simulink model "L1HeadingController"  (R2015a)
settings: Solver=ode4  StartTime=0.0  StopTime=10.0  FixedStep=0.01  RelTol=1e-3
undefined symbols (not defined in the file): a1, a2, delta_rate_limit, Pb_yaw, proj_omega_0_yaw, proj_omega_bound_yaw, proj_omega_center_yaw, proj_omega_eps_yaw, proj_sigma_0_yaw, proj_sigma_bound_yaw, proj_sigma_center_yaw, proj_sigma_eps_yaw, proj_theta_0_yaw, proj_theta_bound_yaw, proj_theta_center_yaw, proj_theta_eps_yaw, T, theta_1, Ts, Ts_yaw_L1
libraries: vrlib x6, simulink x2
settings Model: Creator=s120949  LastModifiedBy=s120949
settings OptimizationCC: OptimizeModelRefInitCode=on  LifeSpan=1
settings RTWCC: SystemTargetFile=ert.tlc  GenCodeOnly=on  TemplateMakefile=ert_default_tmf  Description=Embedded Coder  BuildConfiguration=Faster Runs
settings CodeAppCC: IgnoreCustomStorageClasses=off  SignalNamingRule=Custom
settings ERTTargetCC: ParMdlRefBuildCompliant=on  CompOptLevelCompliant=on  ConcurrentExecutionCompliant=on  ERTFirstTimeCompliant=on  SupportContinuousTime=off  SupportVariableSizeSignals=off  ModelStepFunctionPrototypeControlCompliant=on  CPPClassGenCompliant=on  InlinedParameterPlacement=Hierarchical  ERTCustomFileTemplate=example_file_process.tlc  ConvertIfToSwitch=on

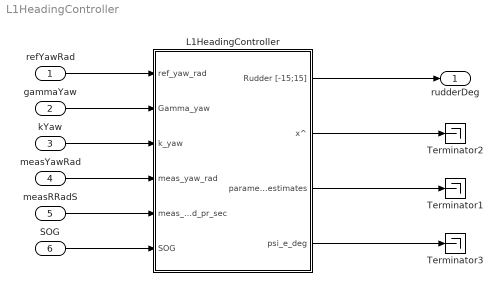
== system L1HeadingController ==
  refYawRad : Inport
  gammaYaw : Inport  Port=2
  kYaw : Inport  Port=3
  measYawRad : Inport  Port=4
  measRRadS : Inport  Port=5
  SOG : Inport  Port=6
  L1HeadingController : Subsystem  TreatAsAtomicUnit=on
      settings: RTWSystemCode=Nonreusable function
  Terminator1 : Terminator
  Terminator2 : Terminator
  Terminator3 : Terminator
  rudderDeg : Outport
  wires:
  refYawRad/1 -> L1HeadingController/1(ref_yaw_rad)
  L1HeadingController/1(Rudder [-15;15]) -> rudderDeg/1
  gammaYaw/1 -> L1HeadingController/2(Gamma_yaw)
  kYaw/1 -> L1HeadingController/3(k_yaw)
  measYawRad/1 -> L1HeadingController/4(meas_yaw_rad)
  measRRadS/1 -> L1HeadingController/5(meas_R_rad_pr_sec)
  SOG/1 -> L1HeadingController/6(SOG)
  L1HeadingController/2(x^) -> Terminator2/1
  L1HeadingController/4(psi_e_deg) -> Terminator3/1
  L1HeadingController/3(parameter_estimates) -> Terminator1/1

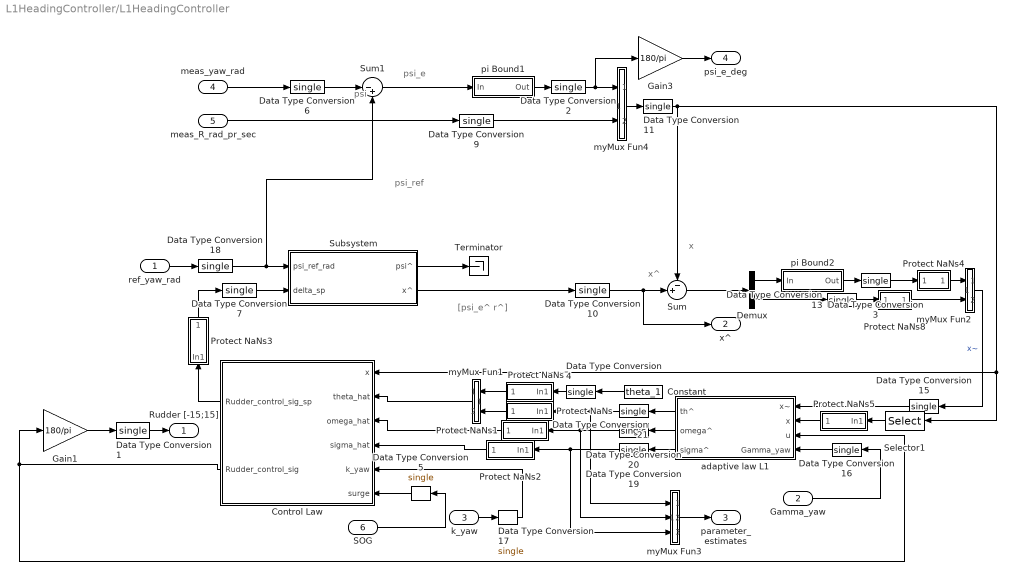
== system L1HeadingController/L1HeadingController ==
  note: x^
  note: [psi_e^ r^]
  note: x
  note: psi
  note: psi_ref
  note: psi_e
  ref_yaw_rad : Inport
  Gamma_yaw : Inport  Port=2
  k_yaw : Inport  Port=3
  meas_yaw_rad : Inport  Port=4
  meas_R_rad_pr_sec : Inport  Port=5
  SOG : Inport  Port=6
  Constant : Constant  Value=theta_1  SampleTime=Ts_yaw_L1
  Control Law : Subsystem
  Data Type Conversion{1..7,9..11,13,15..21} (18 alike) : DataTypeConversion  OutDataTypeStr=single
  Demux : Demux  Outputs=2
  Gain1 : Gain  Gain=180/pi
  Gain3 : Gain  Gain=180/pi
  Protect NaNs : Subsystem
  Protect NaNs1 : Subsystem
  Protect NaNs2 : Subsystem
  Protect NaNs3 : Subsystem
  Protect NaNs4 : Subsystem
  Protect NaNs5 : Subsystem
  Protect NaNs7 : Subsystem
  Protect NaNs8 : Subsystem
  Selector1 : Selector  InputPortWidth=2  Indices=2
  Subsystem : Subsystem
  Sum : Sum  Inputs=-+|
  Sum1 : Sum  Inputs=|-+
  Terminator : Terminator
  adaptive law L1 : Subsystem
  myMux Fun1 : MATLAB Function  TreatAsAtomicUnit=on
  myMux Fun2 : MATLAB Function  TreatAsAtomicUnit=on
  myMux Fun3 : MATLAB Function  TreatAsAtomicUnit=on
  myMux Fun4 : MATLAB Function  TreatAsAtomicUnit=on
  pi Bound1 : Subsystem  AncestorBlock=aerosimlib/Math/pi Bound  mask(pi bound){}
      mask help: Bounds the input angle to [-pi, pi]. When -pi bound is exceeded the output wraps back to pi; when the pi bound is exceeded the output wraps back to -pi.
      mask Help:
      | Bounds the input angle to [-pi, pi]. When -pi bound is exceeded the output wraps back to pi; when the pi bound is exceeded the output wraps back to -pi.
      | <P><B>Input:</B> any angle in radians, from -Inf to Inf;</P>
      | <P><B>Output:</B> an angle in radians between -pi and pi.</P>
  pi Bound2 : Subsystem  AncestorBlock=aerosimlib/Math/pi Bound  mask(pi bound){}
      mask help: Bounds the input angle to [-pi, pi]. When -pi bound is exceeded the output wraps back to pi; when the pi bound is exceeded the output wraps back to -pi.
      mask Help:
      | Bounds the input angle to [-pi, pi]. When -pi bound is exceeded the output wraps back to pi; when the pi bound is exceeded the output wraps back to -pi.
      | <P><B>Input:</B> any angle in radians, from -Inf to Inf;</P>
      | <P><B>Output:</B> an angle in radians between -pi and pi.</P>
  Rudder [-15;15] : Outport
  x^ : Outport  Port=2
  parameter_estimates : Outport  Port=3
  psi_e_deg : Outport  Port=4
  wires:
  Gamma_yaw/1 -> Data Type Conversion16/1
  k_yaw/1 -> Data Type Conversion17/1
  adaptive law L1/3(sigma^) -> Data Type Conversion19/1
  adaptive law L1/2(omega^) -> Data Type Conversion20/1
  ref_yaw_rad/1 -> Data Type Conversion18/1
  Control Law/2(Rudder_control_sig) -> adaptive law L1/3(u), Gain1/1
  adaptive law L1/1(th^) -> Data Type Conversion21/1
  Control Law/1(Rudder_control_sig_sp) -> Protect NaNs3/1(In1)
  meas_yaw_rad/1 -> Data Type Conversion6/1
  meas_R_rad_pr_sec/1 -> Data Type Conversion9/1
  Sum/1 -> Demux/1
  Demux/1 -> pi Bound2/1(In)
  Demux/2 -> Data Type Conversion13/1
  pi Bound2/1(Out) -> Data Type Conversion3/1
  myMux Fun2/1(y) -> Data Type Conversion15/1  "x~"
  Subsystem/2(x^) -> Data Type Conversion10/1
  pi Bound1/1(Out) -> Data Type Conversion2/1
  myMux Fun4/1(y) -> Data Type Conversion11/1
  Sum1/1 -> pi Bound1/1(In)
  Subsystem/1(psi^) -> Terminator/1
  Data Type Conversion1/1 -> Rudder [-15;15]/1
  Data Type Conversion6/1 -> Sum1/1
  Data Type Conversion9/1 -> myMux Fun4/2(u2)
  Data Type Conversion10/1 -> Sum/2, x^/1
  Data Type Conversion11/1 -> Sum/1, Control Law/1(x), Selector1/1
  Data Type Conversion13/1 -> Protect NaNs8/1(In1)
  Data Type Conversion15/1 -> adaptive law L1/1(x~)
  Data Type Conversion16/1 -> adaptive law L1/4(Gamma_yaw)
  Data Type Conversion17/1 -> Control Law/5(k_yaw)
  Data Type Conversion18/1 -> Subsystem/1(psi_ref_rad), Sum1/2
  Data Type Conversion7/1 -> Subsystem/2(delta_sp)
  Data Type Conversion19/1 -> myMux Fun3/3(u3), Protect NaNs2/1(In1)
  Data Type Conversion20/1 -> myMux Fun3/2(u2), Protect NaNs1/1(In1)
  Data Type Conversion2/1 -> myMux Fun4/1(u1), Gain3/1
  Gain3/1 -> psi_e_deg/1
  Gain1/1 -> Data Type Conversion1/1
  Selector1/1 -> Protect NaNs5/1(In1)
  Data Type Conversion21/1 -> myMux Fun3/1(u1), Protect NaNs/1(In1)
  Data Type Conversion4/1 -> Protect NaNs7/1(In1)
  myMux Fun1/1(y) -> Control Law/2(theta_hat)
  Constant/1 -> Data Type Conversion4/1
  myMux Fun3/1(y) -> parameter_estimates/1
  Protect NaNs/1(Out1) -> myMux Fun1/2(u2)
  Protect NaNs1/1(Out1) -> Control Law/3(omega_hat)
  Protect NaNs2/1(Out1) -> Control Law/4(sigma_hat)
  Protect NaNs3/1(Out1) -> Data Type Conversion7/1
  Protect NaNs7/1(Out1) -> myMux Fun1/1(u1)
  Protect NaNs5/1(Out1) -> adaptive law L1/2(x)
  Protect NaNs4/1(Out1) -> myMux Fun2/1(u1)
  Protect NaNs8/1(Out1) -> myMux Fun2/2(u2)
  Data Type Conversion3/1 -> Protect NaNs4/1(In1)
  Data Type Conversion5/1 -> Control Law/6(surge)
  SOG/1 -> Data Type Conversion5/1

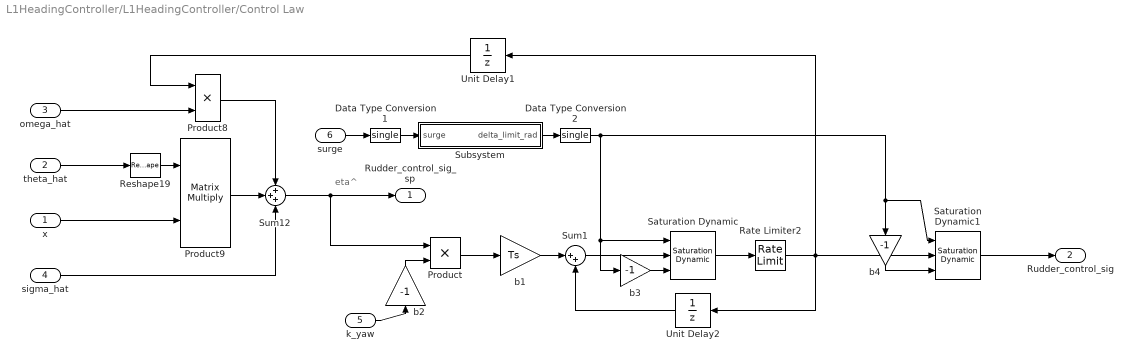
== system L1HeadingController/L1HeadingController/Control Law ==
  note: eta^
  x : Inport
  theta_hat : Inport  Port=2
  omega_hat : Inport  Port=3
  sigma_hat : Inport  Port=4
  k_yaw : Inport  Port=5
  surge : Inport  Port=6
  Data Type Conversion1 : DataTypeConversion  OutDataTypeStr=single
  Data Type Conversion2 : DataTypeConversion  OutDataTypeStr=single
  Product : Product  RndMeth=Zero
  Product8 : Product  RndMeth=Zero
  Product9 : Product  Multiplication=Matrix(*)  RndMeth=Zero
  Rate Limiter2 : RateLimiter  RisingSlewLimit=delta_rate_limit  FallingSlewLimit=-delta_rate_limit  SampleTimeMode=inherited
  Reshape19 : Reshape  OutputDimensionality=Row vector (2-D)
  Saturation Dynamic : simulink/Discontinuities/Saturation Dynamic  OutMin=[]  OutMax=[]  OutDataTypeStr=Inherit: Same as second input  OutDataType=fixdt(1, 16)  OutScaling=2^-10  DoSatur=off
  Saturation Dynamic1 : simulink/Discontinuities/Saturation Dynamic  OutMin=[]  OutMax=[]  OutDataTypeStr=Inherit: Same as second input  OutDataType=fixdt(1, 16)  OutScaling=2^-10  DoSatur=off
  Subsystem : Subsystem
  Sum1 : Sum  Inputs=|++
  Sum12 : Sum  Inputs=+++
  Unit Delay1 : UnitDelay  SampleTime=Ts
  Unit Delay2 : UnitDelay  SampleTime=Ts
  b1 : Gain  Gain=Ts  SampleTime=Ts
  b2 : Gain  Gain=-1
  b3 : Gain  Gain=-1
  b4 : Gain  Gain=-1
  Rudder_control_sig_sp : Outport
  Rudder_control_sig : Outport  Port=2
  wires:
  k_yaw/1 -> b2/1
  b2/1 -> Product/2
  Unit Delay1/1 -> Product8/1
  Product/1 -> b1/1
  Sum12/1 -> Rudder_control_sig_sp/1, Product/1
  sigma_hat/1 -> Sum12/3
  Product8/1 -> Sum12/1
  Product9/1 -> Sum12/2
  x/1 -> Product9/2
  Reshape19/1 -> Product9/1
  theta_hat/1 -> Reshape19/1
  omega_hat/1 -> Product8/2
  Sum1/1 -> Saturation Dynamic/2
  Saturation Dynamic/1 -> Rate Limiter2/1
  b1/1 -> Sum1/1
  Subsystem/1(delta_limit_rad) -> Data Type Conversion2/1
  b3/1 -> Saturation Dynamic/3
  surge/1 -> Data Type Conversion1/1
  Rate Limiter2/1 -> Unit Delay1/1, Saturation Dynamic1/2, Unit Delay2/1
  Unit Delay2/1 -> Sum1/2
  Saturation Dynamic1/1 -> Rudder_control_sig/1
  b4/1 -> Saturation Dynamic1/3
  Data Type Conversion1/1 -> Subsystem/1(surge)
  Data Type Conversion2/1 -> Saturation Dynamic/1, b3/1, Saturation Dynamic1/1, b4/1

== system L1HeadingController/L1HeadingController/Protect NaNs ==
  In1 : Inport
  Integer Delay3 : Delay  DelayLength=1  InputProcessing=Inherited  SampleTime=T
  Relational Operator2 : RelationalOperator  Operator===  OutDataTypeStr=uint(8)
  Switch3 : Switch  Criteria=u2 > Threshold  Threshold=0.3  SampleTime=.01
  Out1 : Outport
  wires:
  Integer Delay3/1 -> Switch3/3
  Switch3/1 -> Out1/1, Integer Delay3/1
  In1/1 -> Relational Operator2/2, Relational Operator2/1, Switch3/1
  Relational Operator2/1 -> Switch3/2

== system L1HeadingController/L1HeadingController/Protect NaNs1 ==
  In1 : Inport
  Integer Delay3 : Delay  DelayLength=1  InputProcessing=Inherited  SampleTime=T
  Relational Operator2 : RelationalOperator  Operator===  OutDataTypeStr=uint(8)
  Switch3 : Switch  Criteria=u2 > Threshold  Threshold=0.3  SampleTime=.01
  Out1 : Outport
  wires:
  Relational Operator2/1 -> Switch3/2
  In1/1 -> Switch3/1, Relational Operator2/1, Relational Operator2/2
  Switch3/1 -> Integer Delay3/1, Out1/1
  Integer Delay3/1 -> Switch3/3

== system L1HeadingController/L1HeadingController/Protect NaNs2 ==
  In1 : Inport
  Integer Delay3 : Delay  DelayLength=1  InputProcessing=Inherited  SampleTime=T
  Relational Operator2 : RelationalOperator  Operator===  OutDataTypeStr=uint(8)
  Switch3 : Switch  Criteria=u2 > Threshold  Threshold=0.3  SampleTime=.01
  Out1 : Outport
  wires:
  Integer Delay3/1 -> Switch3/3
  Switch3/1 -> Out1/1, Integer Delay3/1
  In1/1 -> Relational Operator2/2, Relational Operator2/1, Switch3/1
  Relational Operator2/1 -> Switch3/2

== system L1HeadingController/L1HeadingController/Protect NaNs3 ==
  In1 : Inport
  Integer Delay3 : Delay  DelayLength=1  InputProcessing=Inherited  SampleTime=T
  Relational Operator2 : RelationalOperator  Operator===  OutDataTypeStr=uint(8)
  Switch3 : Switch  Criteria=u2 > Threshold  Threshold=0.3  SampleTime=.01
  Out1 : Outport
  wires:
  Relational Operator2/1 -> Switch3/2
  In1/1 -> Switch3/1, Relational Operator2/1, Relational Operator2/2
  Switch3/1 -> Integer Delay3/1, Out1/1
  Integer Delay3/1 -> Switch3/3

== system L1HeadingController/L1HeadingController/Protect NaNs4 ==
  In1 : Inport
  Integer Delay3 : Delay  DelayLength=1  InputProcessing=Inherited  SampleTime=T
  Relational Operator2 : RelationalOperator  Operator===  OutDataTypeStr=uint(8)
  Switch3 : Switch  Criteria=u2 > Threshold  Threshold=0.3  SampleTime=.01
  Out1 : Outport
  wires:
  Integer Delay3/1 -> Switch3/3
  Switch3/1 -> Out1/1, Integer Delay3/1
  In1/1 -> Relational Operator2/2, Relational Operator2/1, Switch3/1
  Relational Operator2/1 -> Switch3/2

== system L1HeadingController/L1HeadingController/Protect NaNs5 ==
  In1 : Inport
  Integer Delay3 : Delay  DelayLength=1  InputProcessing=Inherited  SampleTime=T
  Relational Operator2 : RelationalOperator  Operator===  OutDataTypeStr=uint(8)
  Switch3 : Switch  Criteria=u2 > Threshold  Threshold=0.3  SampleTime=.01
  Out1 : Outport
  wires:
  Relational Operator2/1 -> Switch3/2
  In1/1 -> Switch3/1, Relational Operator2/1, Relational Operator2/2
  Switch3/1 -> Integer Delay3/1, Out1/1
  Integer Delay3/1 -> Switch3/3

== system L1HeadingController/L1HeadingController/Protect NaNs7 ==
  In1 : Inport
  Integer Delay3 : Delay  DelayLength=1  InputProcessing=Inherited  SampleTime=T
  Relational Operator2 : RelationalOperator  Operator===  OutDataTypeStr=uint(8)
  Switch3 : Switch  Criteria=u2 > Threshold  Threshold=0.3  SampleTime=.01
  Out1 : Outport
  wires:
  Relational Operator2/1 -> Switch3/2
  In1/1 -> Switch3/1, Relational Operator2/1, Relational Operator2/2
  Switch3/1 -> Integer Delay3/1, Out1/1
  Integer Delay3/1 -> Switch3/3

== system L1HeadingController/L1HeadingController/Protect NaNs8 ==
  In1 : Inport
  Integer Delay3 : Delay  DelayLength=1  InputProcessing=Inherited  SampleTime=T
  Relational Operator2 : RelationalOperator  Operator===  OutDataTypeStr=uint(8)
  Switch3 : Switch  Criteria=u2 > Threshold  Threshold=0.3  SampleTime=.01
  Out1 : Outport
  wires:
  Relational Operator2/1 -> Switch3/2
  In1/1 -> Switch3/1, Relational Operator2/1, Relational Operator2/2
  Switch3/1 -> Integer Delay3/1, Out1/1
  Integer Delay3/1 -> Switch3/3

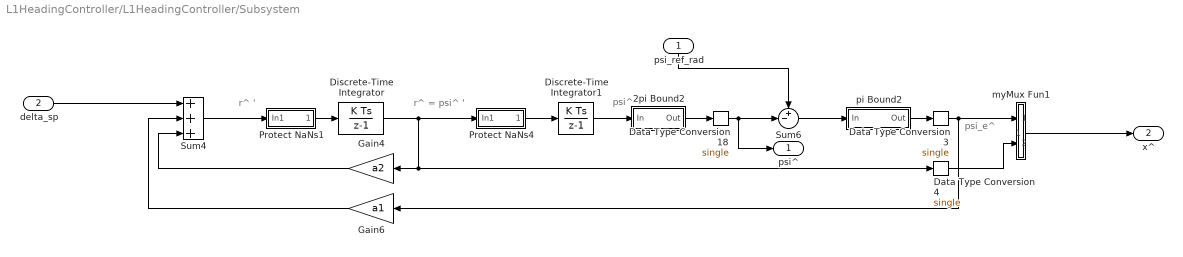
== system L1HeadingController/L1HeadingController/Subsystem ==
  note: r^ '
  note: r^ = psi^ '
  note: psi^
  note: psi_e^
  psi_ref_rad : Inport
  delta_sp : Inport  Port=2
  2pi Bound2 : Subsystem  AncestorBlock=aerosimlib/Math/2pi Bound  mask(2pi bound){}
      mask help: Bounds the input angle to [0, 2pi]. When 0 bound is exceeded the output wraps back to 2pi; when the 2pi bound is exceeded the output wraps back to 0.
      mask Help:
      | Bounds the input angle to [0, 2pi]. When 0 bound is exceeded the output wraps back to 2pi; when the 2pi bound is exceeded the output wraps back to 0.
      | <P><B>Input:</B> any angle in radians, from -Inf to Inf;</P>
      | <P><B>Output:</B> an angle in radians between zero and 2pi.</P>
  Data Type Conversion18 : DataTypeConversion  OutDataTypeStr=single
  Data Type Conversion3 : DataTypeConversion  OutDataTypeStr=single
  Data Type Conversion4 : DataTypeConversion  OutDataTypeStr=single
  Discrete-Time Integrator : DiscreteIntegrator  SampleTime=Ts_yaw_L1  LimitOutput=on  UpperSaturationLimit=pi/2  LowerSaturationLimit=-pi/2
  Discrete-Time Integrator1 : DiscreteIntegrator  SampleTime=Ts_yaw_L1
  Gain4 : Gain  Gain=a2
  Gain6 : Gain  Gain=a1
  Protect NaNs1 : Subsystem
  Protect NaNs4 : Subsystem
  Sum4 : Sum  Inputs=+++
  Sum6 : Sum  Inputs=+-|
  myMux Fun1 : MATLAB Function  TreatAsAtomicUnit=on
  pi Bound2 : Subsystem  AncestorBlock=aerosimlib/Math/pi Bound  mask(pi bound){}
      mask help: Bounds the input angle to [-pi, pi]. When -pi bound is exceeded the output wraps back to pi; when the pi bound is exceeded the output wraps back to -pi.
      mask Help:
      | Bounds the input angle to [-pi, pi]. When -pi bound is exceeded the output wraps back to pi; when the pi bound is exceeded the output wraps back to -pi.
      | <P><B>Input:</B> any angle in radians, from -Inf to Inf;</P>
      | <P><B>Output:</B> an angle in radians between -pi and pi.</P>
  psi^ : Outport
  x^ : Outport  Port=2
  wires:
  Discrete-Time Integrator/1 -> Gain4/1, Data Type Conversion4/1, Protect NaNs4/1(In1)
  Sum4/1 -> Protect NaNs1/1(In1)
  Discrete-Time Integrator1/1 -> 2pi Bound2/1(In)
  Gain4/1 -> Sum4/3
  Gain6/1 -> Sum4/2
  psi_ref_rad/1 -> Sum6/1
  delta_sp/1 -> Sum4/1
  myMux Fun1/1(y) -> x^/1
  pi Bound2/1(Out) -> Data Type Conversion3/1
  2pi Bound2/1(Out) -> Data Type Conversion18/1
  Data Type Conversion18/1 -> Sum6/2, psi^/1
  Sum6/1 -> pi Bound2/1(In)
  Data Type Conversion3/1 -> Gain6/1, myMux Fun1/1(u1)
  Data Type Conversion4/1 -> myMux Fun1/2(u2)
  Protect NaNs4/1(Out1) -> Discrete-Time Integrator1/1
  Protect NaNs1/1(Out1) -> Discrete-Time Integrator/1

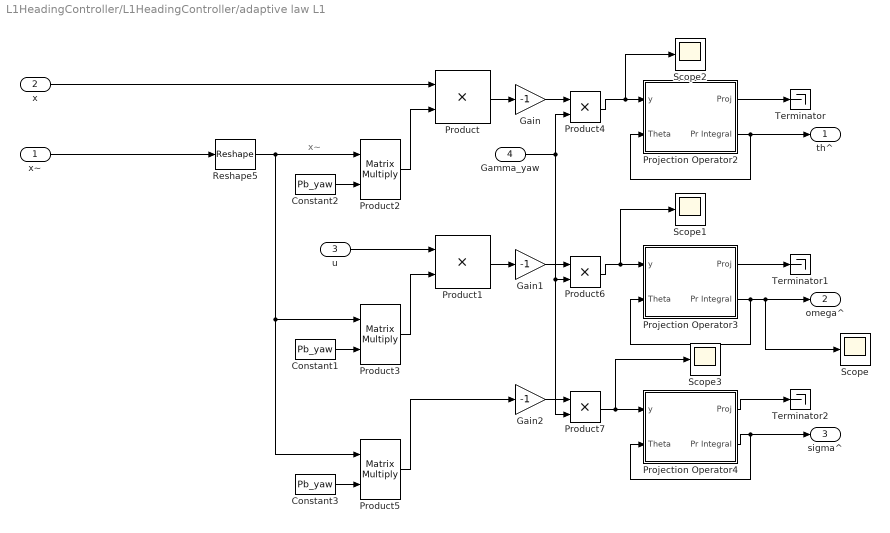
== system L1HeadingController/L1HeadingController/adaptive law L1 ==
  note: x~
  x~ : Inport
  x : Inport  Port=2
  u : Inport  Port=3
  Gamma_yaw : Inport  Port=4
  Constant1 : Constant  Value=Pb_yaw  SampleTime=Ts_yaw_L1
  Constant2 : Constant  Value=Pb_yaw  SampleTime=Ts_yaw_L1
  Constant3 : Constant  Value=Pb_yaw  SampleTime=Ts_yaw_L1
  Gain : Gain  Gain=-1
  Gain1 : Gain  Gain=-1
  Gain2 : Gain  Gain=-1
  Product{,1,4,6..7} (5 alike) : Product  RndMeth=Zero
  Product2 : Product  Multiplication=Matrix(*)  RndMeth=Zero
  Product3 : Product  Multiplication=Matrix(*)  RndMeth=Zero
  Product5 : Product  Multiplication=Matrix(*)  RndMeth=Zero
  Projection Operator2 : Subsystem  AncestorBlock=Projection/Projection Operator  mask{EpsilonTheta=proj_theta_eps_yaw, Prmax=proj_theta_bound_yaw, Prcenter=proj_theta_center_yaw, Pr0=proj_theta_0_yaw}
      mask prompts: EpsilonTheta "Epsilon"; Prmax "Bound (radius of the ball)"; Prcenter "Center of the Ball"; Pr0 "Initialization of integral"
      mask help:
      | Computes projection of the signal and safely integrate it.
      | Works both for scalar and vector signals.
      | It considers the parameter set as a ball at the specified location with
      | preset radius.
      mask init:
      | Thetamax = Prmax / sqrt(EpsilonTheta+1);
      | Intmax = Prmax+Prcenter;
      | Intmin = -Prmax+Prcenter;
  Projection Operator3 : Subsystem  AncestorBlock=Projection/Projection Operator  mask{EpsilonTheta=proj_omega_eps_yaw, Prmax=proj_omega_bound_yaw, Prcenter=proj_omega_center_yaw, Pr0=proj_omega_0_yaw}
      mask prompts: EpsilonTheta "Epsilon"; Prmax "Bound (radius of the ball)"; Prcenter "Center of the Ball"; Pr0 "Initialization of integral"
      mask help:
      | Computes projection of the signal and safely integrate it.
      | Works both for scalar and vector signals.
      | It considers the parameter set as a ball at the specified location with
      | preset radius.
      mask init:
      | Thetamax = Prmax / sqrt(EpsilonTheta+1);
      | Intmax = Prmax+Prcenter;
      | Intmin = -Prmax+Prcenter;
  Projection Operator4 : Subsystem  AncestorBlock=Projection/Projection Operator  mask{EpsilonTheta=proj_sigma_eps_yaw, Prmax=proj_sigma_bound_yaw, Prcenter=proj_sigma_center_yaw, Pr0=proj_sigma_0_yaw}
      mask prompts: EpsilonTheta "Epsilon"; Prmax "Bound (radius of the ball)"; Prcenter "Center of the Ball"; Pr0 "Initialization of integral"
      mask help:
      | Computes projection of the signal and safely integrate it.
      | Works both for scalar and vector signals.
      | It considers the parameter set as a ball at the specified location with
      | preset radius.
      mask init:
      | Thetamax = Prmax / sqrt(EpsilonTheta+1);
      | Intmax = Prmax+Prcenter;
      | Intmin = -Prmax+Prcenter;
  Reshape5 : Reshape  OutputDimensionality=Row vector (2-D)
  Scope{,1..3} (4 alike) : Scope
      Scope settings: SaveName=ScopeData7
      Scope1 settings: SaveName=ScopeData8
      Scope2 settings: SaveName=ScopeData9
      Scope3 settings: SaveName=ScopeData10
  Terminator : Terminator
  Terminator1 : Terminator
  Terminator2 : Terminator
  th^ : Outport
  omega^ : Outport  Port=2
  sigma^ : Outport  Port=3
  wires:
  Gamma_yaw/1 -> Product7/2, Product6/2, Product4/2
  Gain2/1 -> Product7/1
  Gain1/1 -> Product6/1
  Gain/1 -> Product4/1
  u/1 -> Product1/1
  Projection Operator4/1(Proj) -> Terminator2/1
  Projection Operator4/2(Pr Integral) -> Projection Operator4/2(Theta), sigma^/1
  Constant3/1 -> Product5/2
  Product5/1 -> Gain2/1
  Product7/1 -> Scope3/1, Projection Operator4/1(y)
  Projection Operator3/1(Proj) -> Terminator1/1
  Projection Operator3/2(Pr Integral) -> Scope/1, omega^/1, Projection Operator3/2(Theta)
  Constant1/1 -> Product3/2
  Product3/1 -> Product1/2
  Product1/1 -> Gain1/1
  Product6/1 -> Scope1/1, Projection Operator3/1(y)
  Projection Operator2/1(Proj) -> Terminator/1
  Projection Operator2/2(Pr Integral) -> Projection Operator2/2(Theta), th^/1
  Reshape5/1 -> Product5/1, Product3/1, Product2/1
  Constant2/1 -> Product2/2
  Product2/1 -> Product/2
  x~/1 -> Reshape5/1
  x/1 -> Product/1
  Product/1 -> Gain/1
  Product4/1 -> Scope2/1, Projection Operator2/1(y)

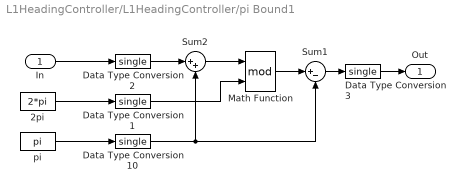
== system L1HeadingController/L1HeadingController/pi Bound1 ==
  In : Inport
  2pi : Constant  Value=2*pi
  Data Type Conversion{1..3,10} (4 alike) : DataTypeConversion  OutDataTypeStr=single
  Math Function : Math  Operator=mod  SaturateOnIntegerOverflow=on
  Sum1 : Sum  Inputs=|+-  SaturateOnIntegerOverflow=on  InputSameDT=on  OutDataTypeStr=Inherit: Same as first input
  Sum2 : Sum  Inputs=|++  SaturateOnIntegerOverflow=on  InputSameDT=on  OutDataTypeStr=Inherit: Same as first input
  pi : Constant  Value=pi
  Out : Outport
  wires:
  Sum1/1 -> Data Type Conversion3/1
  pi/1 -> Data Type Conversion10/1
  Sum2/1 -> Math Function/1
  In/1 -> Data Type Conversion2/1
  2pi/1 -> Data Type Conversion1/1
  Math Function/1 -> Sum1/1
  Data Type Conversion10/1 -> Sum1/2, Sum2/2
  Data Type Conversion1/1 -> Math Function/2
  Data Type Conversion2/1 -> Sum2/1
  Data Type Conversion3/1 -> Out/1

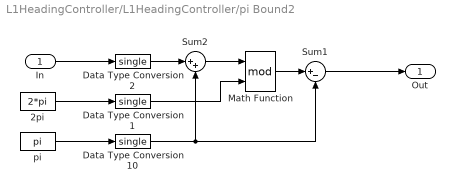
== system L1HeadingController/L1HeadingController/pi Bound2 ==
  In : Inport
  2pi : Constant  Value=2*pi
  Data Type Conversion1 : DataTypeConversion  OutDataTypeStr=single
  Data Type Conversion10 : DataTypeConversion  OutDataTypeStr=single
  Data Type Conversion2 : DataTypeConversion  OutDataTypeStr=single
  Math Function : Math  Operator=mod  SaturateOnIntegerOverflow=on
  Sum1 : Sum  Inputs=|+-  SaturateOnIntegerOverflow=on  InputSameDT=on  OutDataTypeStr=Inherit: Same as first input
  Sum2 : Sum  Inputs=|++  SaturateOnIntegerOverflow=on  InputSameDT=on  OutDataTypeStr=Inherit: Same as first input
  pi : Constant  Value=pi
  Out : Outport
  wires:
  Data Type Conversion2/1 -> Sum2/1
  Data Type Conversion1/1 -> Math Function/2
  Data Type Conversion10/1 -> Sum2/2, Sum1/2
  Math Function/1 -> Sum1/1
  2pi/1 -> Data Type Conversion1/1
  In/1 -> Data Type Conversion2/1
  Sum2/1 -> Math Function/1
  pi/1 -> Data Type Conversion10/1
  Sum1/1 -> Out/1

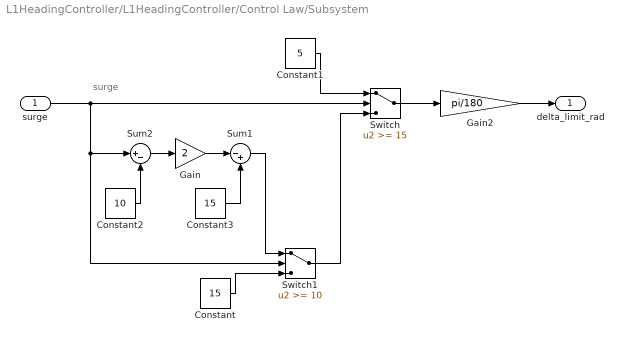
== system L1HeadingController/L1HeadingController/Control Law/Subsystem ==
  note: surge
  surge : Inport
  Constant : Constant  Value=15
  Constant1 : Constant  Value=5
  Constant2 : Constant  Value=10
  Constant3 : Constant  Value=15
  Gain : Gain  Gain=2
  Gain2 : Gain  Gain=pi/180
  Sum1 : Sum  Inputs=|-+
  Sum2 : Sum  Inputs=|+-
  Switch : Switch  Threshold=15
  Switch1 : Switch  Threshold=10
  delta_limit_rad : Outport
  wires:
  surge/1 -> Sum2/1, Switch1/2, Switch/2
  Constant1/1 -> Switch/1
  Switch/1 -> Gain2/1
  Switch1/1 -> Switch/3
  Constant/1 -> Switch1/3
  Sum2/1 -> Gain/1
  Constant2/1 -> Sum2/2
  Gain/1 -> Sum1/1
  Sum1/1 -> Switch1/1
  Constant3/1 -> Sum1/2
  Gain2/1 -> delta_limit_rad/1

== system L1HeadingController/L1HeadingController/Subsystem/2pi Bound2 ==
  In : Inport
  2pi : Constant  Value=2*pi
  Data Type Conversion1 : DataTypeConversion  OutDataTypeStr=single
  Data Type Conversion2 : DataTypeConversion  OutDataTypeStr=single
  Data Type Conversion4 : DataTypeConversion  OutDataTypeStr=single
  Math Function : Math  Operator=mod  SaturateOnIntegerOverflow=on
  Out : Outport
  wires:
  Math Function/1 -> Data Type Conversion4/1
  2pi/1 -> Data Type Conversion2/1
  In/1 -> Data Type Conversion1/1
  Data Type Conversion4/1 -> Out/1
  Data Type Conversion1/1 -> Math Function/1
  Data Type Conversion2/1 -> Math Function/2

== system L1HeadingController/L1HeadingController/Subsystem/Protect NaNs1 ==
  In1 : Inport
  Integer Delay3 : Delay  DelayLength=1  InputProcessing=Inherited  SampleTime=T
  Relational Operator2 : RelationalOperator  Operator===  OutDataTypeStr=uint(8)
  Switch3 : Switch  Criteria=u2 > Threshold  Threshold=0.3  SampleTime=.01
  Out1 : Outport
  wires:
  Relational Operator2/1 -> Switch3/2
  In1/1 -> Switch3/1, Relational Operator2/1, Relational Operator2/2
  Switch3/1 -> Integer Delay3/1, Out1/1
  Integer Delay3/1 -> Switch3/3

== system L1HeadingController/L1HeadingController/Subsystem/Protect NaNs4 ==
  In1 : Inport
  Integer Delay3 : Delay  DelayLength=1  InputProcessing=Inherited  SampleTime=T
  Relational Operator2 : RelationalOperator  Operator===  OutDataTypeStr=uint(8)
  Switch3 : Switch  Criteria=u2 > Threshold  Threshold=0.3  SampleTime=.01
  Out1 : Outport
  wires:
  Integer Delay3/1 -> Switch3/3
  Switch3/1 -> Out1/1, Integer Delay3/1
  In1/1 -> Relational Operator2/2, Relational Operator2/1, Switch3/1
  Relational Operator2/1 -> Switch3/2

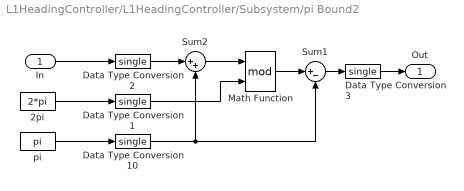
== system L1HeadingController/L1HeadingController/Subsystem/pi Bound2 ==
  In : Inport
  2pi : Constant  Value=2*pi
  Data Type Conversion{1..3,10} (4 alike) : DataTypeConversion  OutDataTypeStr=single
  Math Function : Math  Operator=mod  SaturateOnIntegerOverflow=on
  Sum1 : Sum  Inputs=|+-  SaturateOnIntegerOverflow=on  InputSameDT=on  OutDataTypeStr=Inherit: Same as first input
  Sum2 : Sum  Inputs=|++  SaturateOnIntegerOverflow=on  InputSameDT=on  OutDataTypeStr=Inherit: Same as first input
  pi : Constant  Value=pi
  Out : Outport
  wires:
  Sum1/1 -> Data Type Conversion3/1
  pi/1 -> Data Type Conversion10/1
  Sum2/1 -> Math Function/1
  In/1 -> Data Type Conversion2/1
  2pi/1 -> Data Type Conversion1/1
  Math Function/1 -> Sum1/1
  Data Type Conversion10/1 -> Sum1/2, Sum2/2
  Data Type Conversion1/1 -> Math Function/2
  Data Type Conversion2/1 -> Sum2/1
  Data Type Conversion3/1 -> Out/1

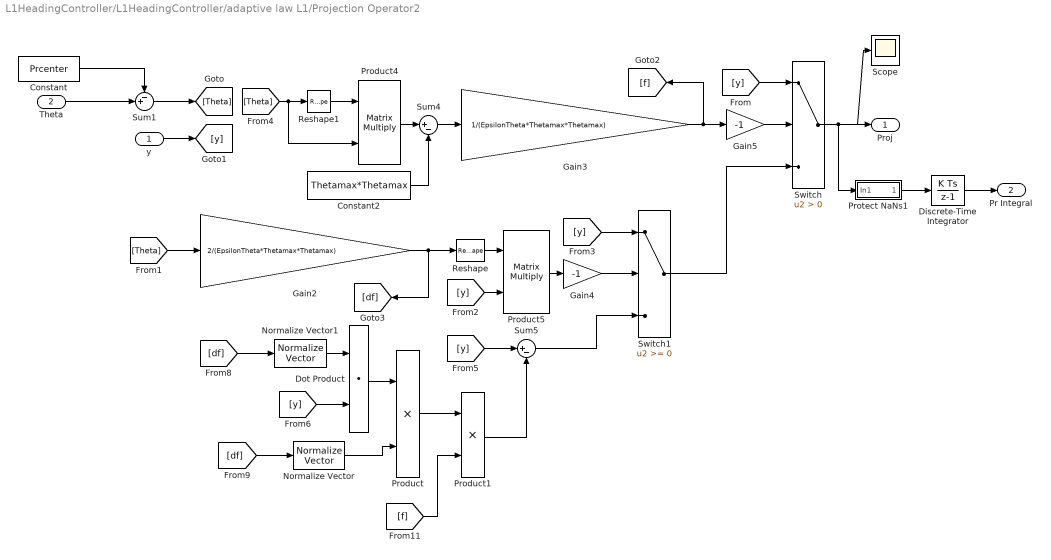
== system L1HeadingController/L1HeadingController/adaptive law L1/Projection Operator2 ==
  y : Inport
  Theta : Inport  Port=2
  Constant : Constant  Value=Prcenter
  Constant2 : Constant  Value=Thetamax*Thetamax
  Discrete-Time Integrator : DiscreteIntegrator  InitialCondition=Pr0  SampleTime=Ts_yaw_L1  LimitOutput=on  UpperSaturationLimit=Intmax  LowerSaturationLimit=Intmin
  Dot Product : DotProduct  InputSameDT=on  OutDataTypeStr=Inherit: Inherit via internal rule
  Gain2 : Gain  Gain=2/(EpsilonTheta*Thetamax*Thetamax)
  Gain3 : Gain  Gain=1/(EpsilonTheta*Thetamax*Thetamax)
  Gain4 : Gain  Gain=-1
  Gain5 : Gain  Gain=-1
  Normalize Vector : vrlib/Utilities/Normalize Vector  maxzero=0
  Normalize Vector1 : vrlib/Utilities/Normalize Vector  maxzero=0
  Product : Product  RndMeth=Zero
  Product1 : Product  RndMeth=Zero
  Product4 : Product  Multiplication=Matrix(*)  RndMeth=Zero
  Product5 : Product  Multiplication=Matrix(*)  RndMeth=Zero
  Protect NaNs1 : Subsystem
  Reshape : Reshape  OutputDimensionality=Row vector (2-D)
  Reshape1 : Reshape  OutputDimensionality=Row vector (2-D)
  Scope : Scope
      settings: SaveName=ScopeData11
  Sum1 : Sum  Inputs=-+|
  Sum4 : Sum  Inputs=|+-
  Sum5 : Sum  Inputs=|+-
  Switch : Switch  Criteria=u2 > Threshold
  Switch1 : Switch
  Proj : Outport
  Pr Integral : Outport  Port=2
  wires:
  Gain5/1 -> Switch/2
  Sum5/1 -> Switch1/3
  [y] -> Sum5/1
  y/1 -> [y]
  Switch/1 -> Scope/1, Proj/1, Protect NaNs1/1(In1)
  Switch1/1 -> Switch/3
  [Theta] -> Gain2/1
  [y] -> Switch1/1
  Gain4/1 -> Switch1/2
  Product5/1 -> Gain4/1
  [y] -> Product5/2
  [y] -> Switch/1
  Gain3/1 -> [f], Gain5/1
  Sum4/1 -> Gain3/1
  Constant2/1 -> Sum4/2
  Product4/1 -> Sum4/1
  [Theta] -> Reshape1/1, Product4/2
  Gain2/1 -> Reshape/1, [df]
  Reshape/1 -> Product5/1
  Reshape1/1 -> Product4/1
  [df] -> Normalize Vector1/1
  [df] -> Normalize Vector/1
  Normalize Vector1/1 -> Dot Product/1
  [y] -> Dot Product/2
  Dot Product/1 -> Product/1
  Normalize Vector/1 -> Product/2
  Product/1 -> Product1/1
  [f] -> Product1/2
  Product1/1 -> Sum5/2
  Discrete-Time Integrator/1 -> Pr Integral/1
  Theta/1 -> Sum1/2
  Sum1/1 -> [Theta]
  Constant/1 -> Sum1/1
  Protect NaNs1/1(Out1) -> Discrete-Time Integrator/1

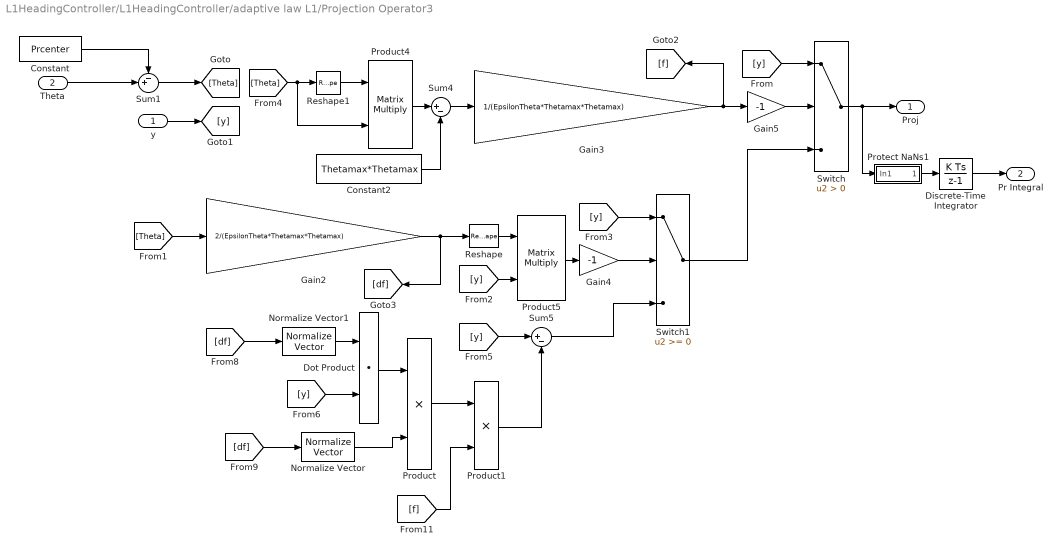
== system L1HeadingController/L1HeadingController/adaptive law L1/Projection Operator3 ==
  y : Inport
  Theta : Inport  Port=2
  Constant : Constant  Value=Prcenter
  Constant2 : Constant  Value=Thetamax*Thetamax
  Discrete-Time Integrator : DiscreteIntegrator  InitialCondition=Pr0  SampleTime=Ts_yaw_L1  LimitOutput=on  UpperSaturationLimit=Intmax  LowerSaturationLimit=Intmin
  Dot Product : DotProduct  InputSameDT=on  OutDataTypeStr=Inherit: Inherit via internal rule
  Gain2 : Gain  Gain=2/(EpsilonTheta*Thetamax*Thetamax)
  Gain3 : Gain  Gain=1/(EpsilonTheta*Thetamax*Thetamax)
  Gain4 : Gain  Gain=-1
  Gain5 : Gain  Gain=-1
  Normalize Vector : vrlib/Utilities/Normalize Vector  maxzero=0
  Normalize Vector1 : vrlib/Utilities/Normalize Vector  maxzero=0
  Product : Product  RndMeth=Zero
  Product1 : Product  RndMeth=Zero
  Product4 : Product  Multiplication=Matrix(*)  RndMeth=Zero
  Product5 : Product  Multiplication=Matrix(*)  RndMeth=Zero
  Protect NaNs1 : Subsystem
  Reshape : Reshape  OutputDimensionality=Row vector (2-D)
  Reshape1 : Reshape  OutputDimensionality=Row vector (2-D)
  Sum1 : Sum  Inputs=-+|
  Sum4 : Sum  Inputs=|+-
  Sum5 : Sum  Inputs=|+-
  Switch : Switch  Criteria=u2 > Threshold
  Switch1 : Switch
  Proj : Outport
  Pr Integral : Outport  Port=2
  wires:
  Constant/1 -> Sum1/1
  Sum1/1 -> [Theta]
  Theta/1 -> Sum1/2
  Discrete-Time Integrator/1 -> Pr Integral/1
  Product1/1 -> Sum5/2
  [f] -> Product1/2
  Product/1 -> Product1/1
  Normalize Vector/1 -> Product/2
  Dot Product/1 -> Product/1
  [y] -> Dot Product/2
  Normalize Vector1/1 -> Dot Product/1
  [df] -> Normalize Vector/1
  [df] -> Normalize Vector1/1
  Reshape1/1 -> Product4/1
  Reshape/1 -> Product5/1
  Gain2/1 -> [df], Reshape/1
  [Theta] -> Product4/2, Reshape1/1
  Product4/1 -> Sum4/1
  Constant2/1 -> Sum4/2
  Sum4/1 -> Gain3/1
  Gain3/1 -> Gain5/1, [f]
  [y] -> Switch/1
  [y] -> Product5/2
  Product5/1 -> Gain4/1
  Gain4/1 -> Switch1/2
  [y] -> Switch1/1
  [Theta] -> Gain2/1
  Switch1/1 -> Switch/3
  Switch/1 -> Proj/1, Protect NaNs1/1(In1)
  y/1 -> [y]
  [y] -> Sum5/1
  Sum5/1 -> Switch1/3
  Gain5/1 -> Switch/2
  Protect NaNs1/1(Out1) -> Discrete-Time Integrator/1

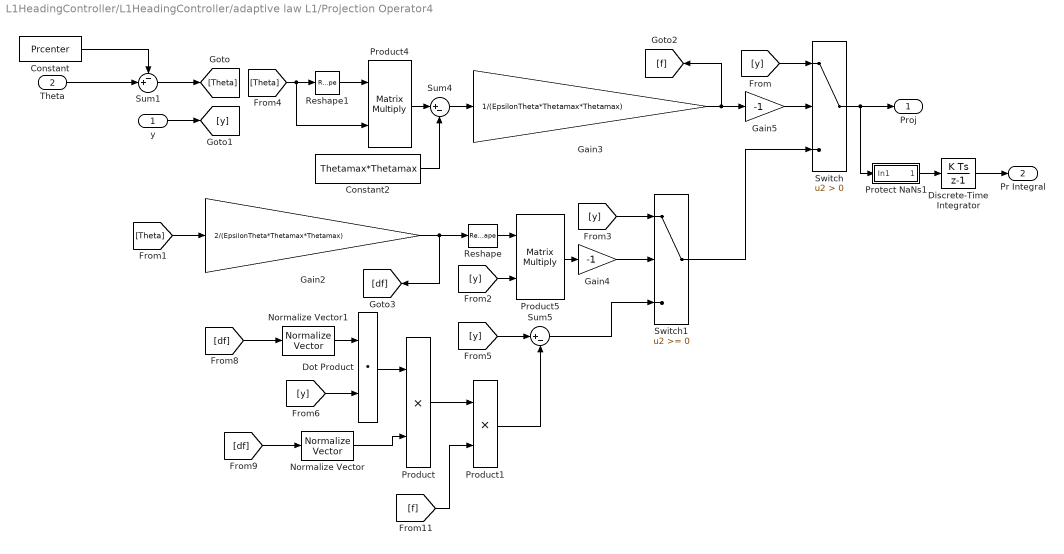
== system L1HeadingController/L1HeadingController/adaptive law L1/Projection Operator4 ==
  y : Inport
  Theta : Inport  Port=2
  Constant : Constant  Value=Prcenter
  Constant2 : Constant  Value=Thetamax*Thetamax
  Discrete-Time Integrator : DiscreteIntegrator  InitialCondition=Pr0  SampleTime=Ts_yaw_L1  LimitOutput=on  UpperSaturationLimit=Intmax  LowerSaturationLimit=Intmin
  Dot Product : DotProduct  InputSameDT=on  OutDataTypeStr=Inherit: Inherit via internal rule
  Gain2 : Gain  Gain=2/(EpsilonTheta*Thetamax*Thetamax)
  Gain3 : Gain  Gain=1/(EpsilonTheta*Thetamax*Thetamax)
  Gain4 : Gain  Gain=-1
  Gain5 : Gain  Gain=-1
  Normalize Vector : vrlib/Utilities/Normalize Vector  maxzero=0
  Normalize Vector1 : vrlib/Utilities/Normalize Vector  maxzero=0
  Product : Product  RndMeth=Zero
  Product1 : Product  RndMeth=Zero
  Product4 : Product  Multiplication=Matrix(*)  RndMeth=Zero
  Product5 : Product  Multiplication=Matrix(*)  RndMeth=Zero
  Protect NaNs1 : Subsystem
  Reshape : Reshape  OutputDimensionality=Row vector (2-D)
  Reshape1 : Reshape  OutputDimensionality=Row vector (2-D)
  Sum1 : Sum  Inputs=-+|
  Sum4 : Sum  Inputs=|+-
  Sum5 : Sum  Inputs=|+-
  Switch : Switch  Criteria=u2 > Threshold
  Switch1 : Switch
  Proj : Outport
  Pr Integral : Outport  Port=2
  wires:
  Constant/1 -> Sum1/1
  Sum1/1 -> [Theta]
  Theta/1 -> Sum1/2
  Discrete-Time Integrator/1 -> Pr Integral/1
  Product1/1 -> Sum5/2
  [f] -> Product1/2
  Product/1 -> Product1/1
  Normalize Vector/1 -> Product/2
  Dot Product/1 -> Product/1
  [y] -> Dot Product/2
  Normalize Vector1/1 -> Dot Product/1
  [df] -> Normalize Vector/1
  [df] -> Normalize Vector1/1
  Reshape1/1 -> Product4/1
  Reshape/1 -> Product5/1
  Gain2/1 -> [df], Reshape/1
  [Theta] -> Product4/2, Reshape1/1
  Product4/1 -> Sum4/1
  Constant2/1 -> Sum4/2
  Sum4/1 -> Gain3/1
  Gain3/1 -> Gain5/1, [f]
  [y] -> Switch/1
  [y] -> Product5/2
  Product5/1 -> Gain4/1
  Gain4/1 -> Switch1/2
  [y] -> Switch1/1
  [Theta] -> Gain2/1
  Switch1/1 -> Switch/3
  Switch/1 -> Proj/1, Protect NaNs1/1(In1)
  y/1 -> [y]
  [y] -> Sum5/1
  Sum5/1 -> Switch1/3
  Gain5/1 -> Switch/2
  Protect NaNs1/1(Out1) -> Discrete-Time Integrator/1

== system L1HeadingController/L1HeadingController/adaptive law L1/Projection Operator2/Protect NaNs1 ==
  In1 : Inport
  Integer Delay3 : Delay  DelayLength=1  InputProcessing=Inherited  SampleTime=T
  Relational Operator2 : RelationalOperator  Operator===  OutDataTypeStr=uint(8)
  Switch3 : Switch  Criteria=u2 > Threshold  Threshold=0.3  SampleTime=.01
  Out1 : Outport
  wires:
  Relational Operator2/1 -> Switch3/2
  In1/1 -> Switch3/1, Relational Operator2/1, Relational Operator2/2
  Switch3/1 -> Integer Delay3/1, Out1/1
  Integer Delay3/1 -> Switch3/3

== system L1HeadingController/L1HeadingController/adaptive law L1/Projection Operator3/Protect NaNs1 ==
  In1 : Inport
  Integer Delay3 : Delay  DelayLength=1  InputProcessing=Inherited  SampleTime=T
  Relational Operator2 : RelationalOperator  Operator===  OutDataTypeStr=uint(8)
  Switch3 : Switch  Criteria=u2 > Threshold  Threshold=0.3  SampleTime=.01
  Out1 : Outport
  wires:
  Relational Operator2/1 -> Switch3/2
  In1/1 -> Switch3/1, Relational Operator2/1, Relational Operator2/2
  Switch3/1 -> Integer Delay3/1, Out1/1
  Integer Delay3/1 -> Switch3/3

== system L1HeadingController/L1HeadingController/adaptive law L1/Projection Operator4/Protect NaNs1 ==
  In1 : Inport
  Integer Delay3 : Delay  DelayLength=1  InputProcessing=Inherited  SampleTime=T
  Relational Operator2 : RelationalOperator  Operator===  OutDataTypeStr=uint(8)
  Switch3 : Switch  Criteria=u2 > Threshold  Threshold=0.3  SampleTime=.01
  Out1 : Outport
  wires:
  Relational Operator2/1 -> Switch3/2
  In1/1 -> Switch3/1, Relational Operator2/1, Relational Operator2/2
  Switch3/1 -> Integer Delay3/1, Out1/1
  Integer Delay3/1 -> Switch3/3

== matlab function L1HeadingController/Subsystem/myMux Fun1 ==
  data: u1 input; y output; u2 input
function y = myMux(u1, u2)
% This block supports an embeddable subset of the MATLAB language.
% See the help menu for details. 

y = [u1(1); u2(1)];

== matlab function L1HeadingController/myMux Fun2 ==
  data: u1 input; y output; u2 input
function y = myMux(u1, u2)
% This block supports an embeddable subset of the MATLAB language.
% See the help menu for details. 

y = [u1(1); u2(1)];

== matlab function L1HeadingController/myMux Fun4 ==
  data: u1 input; y output; u2 input
function y = myMux(u1, u2)
% This block supports an embeddable subset of the MATLAB language.
% See the help menu for details. 

y = [u1(1); u2(1)];

== matlab function L1HeadingController/myMux Fun1 ==
  data: u1 input; y output; u2 input
function y = myMux(u1, u2)
% This block supports an embeddable subset of the MATLAB language.
% See the help menu for details. 

y = [u1(1); u2(1)];

== matlab function L1HeadingController/myMux Fun3 ==
  data: u1 input; y output; u2 input; u3 input
function y = myMux(u1, u2, u3)
% This block supports an embeddable subset of the MATLAB language.
% See the help menu for details. 

y = [u1(1); u2(1); u3(1)];
